simulink model "kurtosis_single_channel_subblocks"  (R2012b)
settings: Solver=ode45  StartTime=0.0  StopTime=3571  RelTol=1e-3
libraries: xbsIndex_r4 x454, xps_library x2, simulink_xsg_bridge x1
(part 1 of 4)
settings Model: Creator=sgowda  LastModifiedBy=sgowda

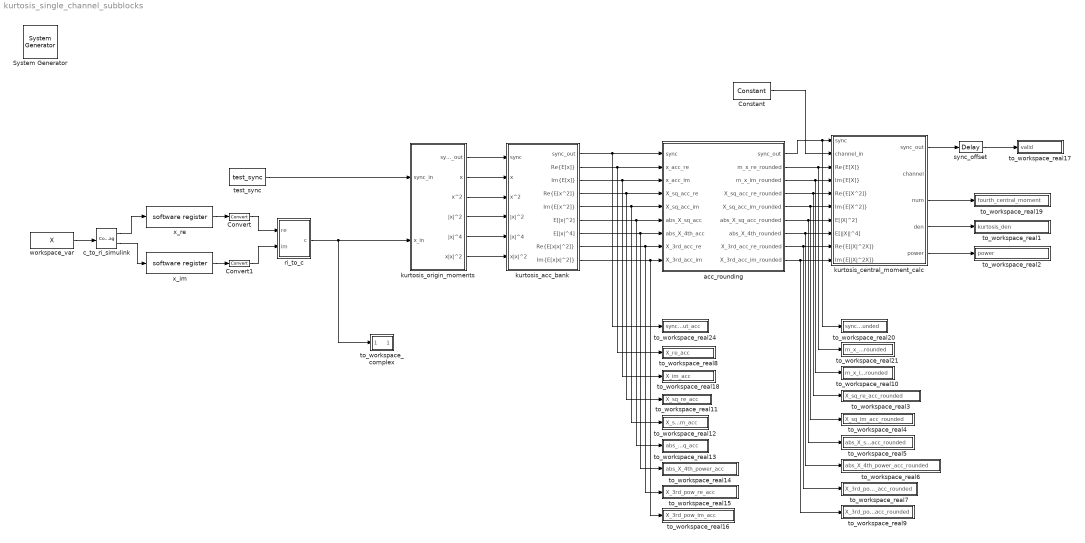
== system kurtosis_single_channel_subblocks ==
  " System Generator" : xbsIndex_r4/ System Generator  Tag=genX  xilinxfamily=Kintex7  part=xc7k325t  speed=-3  package=fbg676  synthesis_tool=XST  clock_wrapper=Clock Enables  directory=./netlist  proj_type=Project Navigator  Synth_file=XST Defaults  Impl_file=ISE Defaults  testbench=off  simulink_period=1  sysclk_period=10  dcm_input_clock_period=10  incr_netlist=off  trim_vbits=Everywhere in SubSystem  dbl_ovrd=According to Block Masks  core_generation=According to Block Masks  run_coregen=off  deprecated_control=off  eval_field=0  block_type=sysgen
  Constant : xbsIndex_r4/Constant  const=0  gui_display_data_type=Fixed-point  arith_type=Signed (2's comp)  n_bits=12  bin_pt=0  preci_type=Single  exp_width=8  frac_width=24  explicit_period=on  period=1  equ=P=C  opselect=C  inp2=PCIN>>17  opr=+  inp1=P  carry=CIN  dbl_ovrd=off  block_type=constant
  Convert : xbsIndex_r4/Convert  gui_display_data_type=Fixed-point  arith_type="Signed  (2's comp)"  n_bits=18  bin_pt=17  float_type=Single  exp_bits=8  fraction_bits=24  quantization=Truncate  overflow=Wrap  en=off  latency=0  dbl_ovrd=off  pipeline=off  block_type=convert
  Convert1 : xbsIndex_r4/Convert  gui_display_data_type=Fixed-point  arith_type="Signed  (2's comp)"  n_bits=18  bin_pt=17  float_type=Single  exp_bits=8  fraction_bits=24  quantization=Truncate  overflow=Wrap  en=off  latency=0  dbl_ovrd=off  pipeline=off  block_type=convert
  acc_rounding : Subsystem
  c_to_ri_simulink : ComplexToRealImag
  kurtosis_acc_bank : Subsystem
  kurtosis_central_moment_calc : Subsystem
  kurtosis_origin_moments : Subsystem
  ri_to_c : Subsystem
  sync_offset : xbsIndex_r4/Delay  rst=off  infoeditControl=Selection of Reset will increase slice count due to use of real FFs and instead of SRLs  en=off  latency=1  dbl_ovrd=off  reg_retiming=off  block_type=delay
  test_sync : simulink_xsg_bridge/test_sync
  to_workspace_complex : Subsystem  mask{var_name=X_fi, n_bits=18, bin_pt=17}
      mask prompts: var_name "Workspace variable name"; n_bits "# of bits"; bin_pt "Binary Point"
      mask init:
      | config.source = str2func('mat_output_data_cplx_init_xblock');
      | config.toplevel = gcb();
      | xBlock(config, {config.toplevel, 'var_name', var_name, ...
      |     'n_bits', n_bits, 'bin_pt', bin_pt});
  to_workspace_real1 : Subsystem  mask{var_name=kurtosis_den}
      mask prompts: var_name "Workspace variable name"
      mask init:
      | %config.source = str2func('mat_output_data_init_xblock');
      | %config.toplevel = gcb();
      | %xBlock(config, {config.toplevel, 'var_name', var_name});
  to_workspace_real10 : Subsystem  mask{var_name=m_x_im_rounded}
      mask prompts: var_name "Workspace variable name"
      mask init:
      | config.source = str2func('mat_output_data_init_xblock');
      | config.toplevel = gcb();
      | xBlock(config, {config.toplevel, 'var_name', var_name});
  to_workspace_real11 : Subsystem  mask{var_name=X_sq_re_acc}
      mask prompts: var_name "Workspace variable name"
      mask init:
      | %config.source = str2func('mat_output_data_init_xblock');
      | %config.toplevel = gcb();
      | %xBlock(config, {config.toplevel, 'var_name', var_name});
  to_workspace_real12 : Subsystem  mask{var_name=X_sq_im_acc}
      mask prompts: var_name "Workspace variable name"
      mask init:
      | %config.source = str2func('mat_output_data_init_xblock');
      | %config.toplevel = gcb();
      | %xBlock(config, {config.toplevel, 'var_name', var_name});
  to_workspace_real13 : Subsystem  mask{var_name=abs_X_sq_acc}
      mask prompts: var_name "Workspace variable name"
      mask init:
      | config.source = str2func('mat_output_data_init_xblock');
      | config.toplevel = gcb();
      | xBlock(config, {config.toplevel, 'var_name', var_name});
  to_workspace_real14 : Subsystem  mask{var_name=abs_X_4th_power_acc}
      mask prompts: var_name "Workspace variable name"
      mask init:
      | %config.source = str2func('mat_output_data_init_xblock');
      | %config.toplevel = gcb();
      | %xBlock(config, {config.toplevel, 'var_name', var_name});
  to_workspace_real15 : Subsystem  mask{var_name=X_3rd_pow_re_acc}
      mask prompts: var_name "Workspace variable name"
      mask init:
      | %config.source = str2func('mat_output_data_init_xblock');
      | %config.toplevel = gcb();
      | %xBlock(config, {config.toplevel, 'var_name', var_name});
  to_workspace_real16 : Subsystem  mask{var_name=X_3rd_pow_im_acc}
      mask prompts: var_name "Workspace variable name"
      mask init:
      | %config.source = str2func('mat_output_data_init_xblock');
      | %config.toplevel = gcb();
      | %xBlock(config, {config.toplevel, 'var_name', var_name});
  to_workspace_real17 : Subsystem  mask{var_name=valid}
      mask prompts: var_name "Workspace variable name"
      mask init:
      | config.source = str2func('mat_output_data_init_xblock');
      | config.toplevel = gcb();
      | xBlock(config, {config.toplevel, 'var_name', var_name});
  to_workspace_real18 : Subsystem  mask{var_name=X_im_acc}
      mask prompts: var_name "Workspace variable name"
      mask init:
      | config.source = str2func('mat_output_data_init_xblock');
      | config.toplevel = gcb();
      | xBlock(config, {config.toplevel, 'var_name', var_name});
  to_workspace_real19 : Subsystem  mask{var_name=fourth_central_moment}
      mask prompts: var_name "Workspace variable name"
      mask init:
      | %config.source = str2func('mat_output_data_init_xblock');
      | %config.toplevel = gcb();
      | %xBlock(config, {config.toplevel, 'var_name', var_name});
  to_workspace_real2 : Subsystem  mask{var_name=power}
      mask prompts: var_name "Workspace variable name"
      mask init:
      | config.source = str2func('mat_output_data_init_xblock');
      | config.toplevel = gcb();
      | xBlock(config, {config.toplevel, 'var_name', var_name});
  to_workspace_real20 : Subsystem  mask{var_name=sync_out_acc_rounded}
      mask prompts: var_name "Workspace variable name"
      mask init:
      | config.source = str2func('mat_output_data_init_xblock');
      | config.toplevel = gcb();
      | xBlock(config, {config.toplevel, 'var_name', var_name});
  to_workspace_real21 : Subsystem  mask{var_name=m_x_re_rounded}
      mask prompts: var_name "Workspace variable name"
      mask init:
      | config.source = str2func('mat_output_data_init_xblock');
      | config.toplevel = gcb();
      | xBlock(config, {config.toplevel, 'var_name', var_name});
  to_workspace_real24 : Subsystem  mask{var_name=sync_out_acc}
      mask prompts: var_name "Workspace variable name"
      mask init:
      | config.source = str2func('mat_output_data_init_xblock');
      | config.toplevel = gcb();
      | xBlock(config, {config.toplevel, 'var_name', var_name});
  to_workspace_real3 : Subsystem  mask{var_name=X_sq_re_acc_rounded}
      mask prompts: var_name "Workspace variable name"
      mask init:
      | config.source = str2func('mat_output_data_init_xblock');
      | config.toplevel = gcb();
      | xBlock(config, {config.toplevel, 'var_name', var_name});
  to_workspace_real4 : Subsystem  mask{var_name=X_sq_im_acc_rounded}
      mask prompts: var_name "Workspace variable name"
      mask init:
      | config.source = str2func('mat_output_data_init_xblock');
      | config.toplevel = gcb();
      | xBlock(config, {config.toplevel, 'var_name', var_name});
  to_workspace_real5 : Subsystem  mask{var_name=abs_X_sq_acc_rounded}
      mask prompts: var_name "Workspace variable name"
      mask init:
      | config.source = str2func('mat_output_data_init_xblock');
      | config.toplevel = gcb();
      | xBlock(config, {config.toplevel, 'var_name', var_name});
  to_workspace_real6 : Subsystem  mask{var_name=abs_X_4th_power_acc_rounded}
      mask prompts: var_name "Workspace variable name"
      mask init:
      | config.source = str2func('mat_output_data_init_xblock');
      | config.toplevel = gcb();
      | xBlock(config, {config.toplevel, 'var_name', var_name});
  to_workspace_real7 : Subsystem  mask{var_name=X_3rd_pow_re_acc_rounded}
      mask prompts: var_name "Workspace variable name"
      mask init:
      | config.source = str2func('mat_output_data_init_xblock');
      | config.toplevel = gcb();
      | xBlock(config, {config.toplevel, 'var_name', var_name});
  to_workspace_real8 : Subsystem  mask{var_name=X_re_acc}
      mask prompts: var_name "Workspace variable name"
      mask init:
      | config.source = str2func('mat_output_data_init_xblock');
      | config.toplevel = gcb();
      | xBlock(config, {config.toplevel, 'var_name', var_name});
  to_workspace_real9 : Subsystem  mask{var_name=X_3rd_pow_im_acc_rounded}
      mask prompts: var_name "Workspace variable name"
      mask init:
      | config.source = str2func('mat_output_data_init_xblock');
      | config.toplevel = gcb();
      | xBlock(config, {config.toplevel, 'var_name', var_name});
  workspace_var : FromWorkspace  VariableName=X  SampleTime=0
  x_im : xps_library/software register  Tag=xps:sw_reg  io_dir=From Processor  arith_type="Signed  (2's comp)"  bitwidth=32  bin_pt=17  sample_period=1  gw_name=kurtosis_single_channel_subblocks_x_im_user_data_out
      link override kurtosis_moment_calc_x_im_user_data_out: arith_type="Signed  (2's comp)"  n_bits=32  bin_pt=17  period=1
      link override untitled3_x_im_user_data_out: gui_display_data_type=Fixed-point  arith_type=Unsigned  n_bits=32  bin_pt=17  preci_type=Single  exp_width=8  frac_width=24  quantization=Truncate  overflow=Wrap  period=1  dbl_ovrd=off  timing_constraint=None  locs_specified=off  LOCs={}  UseAsADC=off  ADCChannel='1'  inherit_from_input=off  hdl_port=on
      link override untitled3_x_im_user_data_out: infoedit="Gateway in block.  Converts inputs of type Simulink integer, single, double and fixed-point to  Xilinx fixed-point or floating-point data type.<br><br>Hardware notes:  In hardware these blocks become top level input ports."
  x_re : xps_library/software register  Tag=xps:sw_reg  io_dir=From Processor  arith_type="Signed  (2's comp)"  bitwidth=32  bin_pt=17  sample_period=1  gw_name=kurtosis_single_channel_subblocks_x_re_user_data_out
      link override untitled3_x_re_user_data_out: gui_display_data_type=Fixed-point  arith_type="Signed  (2's comp)"  n_bits=32  bin_pt=17  preci_type=Single  exp_width=8  frac_width=24  quantization=Truncate  overflow=Wrap  period=1  dbl_ovrd=off  timing_constraint=None  locs_specified=off  LOCs={}  UseAsADC=off  ADCChannel='1'  inherit_from_input=off  hdl_port=on
      link override untitled3_x_re_user_data_out: infoedit="Gateway in block.  Converts inputs of type Simulink integer, single, double and fixed-point to  Xilinx fixed-point or floating-point data type.<br><br>Hardware notes:  In hardware these blocks become top level input ports."
  wires:
  kurtosis_central_moment_calc/1(sync_out) -> sync_offset/1
  sync_offset/1 -> to_workspace_real17/1(valid)
  kurtosis_acc_bank/2("Re{E[x]}") -> to_workspace_real8/1(X_re_acc), acc_rounding/2(x_acc_re)
  kurtosis_acc_bank/3("Im{E[x]}") -> to_workspace_real18/1(X_im_acc), acc_rounding/3(x_acc_im)
  kurtosis_acc_bank/4("Re{E[x^2]}") -> acc_rounding/4(X_sq_acc_re), to_workspace_real11/1(X_sq_re_acc)
  kurtosis_acc_bank/5("Im{E[x^2]}") -> acc_rounding/5(X_sq_acc_im), to_workspace_real12/1(X_sq_im_acc)
  kurtosis_acc_bank/6(E[|x|^2]) -> acc_rounding/6(abs_X_sq_acc), to_workspace_real13/1(abs_X_sq_acc)
  kurtosis_acc_bank/8("Re{E[x|x|^2]}") -> acc_rounding/8(X_3rd_acc_re), to_workspace_real15/1(X_3rd_pow_re_acc)
  kurtosis_acc_bank/7(E[|x|^4]) -> acc_rounding/7(abs_X_4th_acc), to_workspace_real14/1(abs_X_4th_power_acc)
  ri_to_c/1(c) -> kurtosis_origin_moments/2(x_in), to_workspace_complex/1(X_fi)
  Convert/1 -> ri_to_c/1(re)
  Convert1/1 -> ri_to_c/2(im)
  x_im/1 -> Convert1/1
  x_re/1 -> Convert/1
  workspace_var/1 -> c_to_ri_simulink/1
  c_to_ri_simulink/1 -> x_re/1
  c_to_ri_simulink/2 -> x_im/1
  kurtosis_acc_bank/9("Im{E[x|x|^2]}") -> acc_rounding/9(X_3rd_acc_im), to_workspace_real16/1(X_3rd_pow_im_acc)
  kurtosis_acc_bank/1(sync_out) -> acc_rounding/1(sync), to_workspace_real24/1(sync_out_acc)
  test_sync/1 -> kurtosis_origin_moments/1(sync_in)
  kurtosis_origin_moments/1(sync_out) -> kurtosis_acc_bank/1(sync)
  kurtosis_origin_moments/2(x) -> kurtosis_acc_bank/2(x)
  kurtosis_origin_moments/3(x^2) -> kurtosis_acc_bank/3(x^2)
  kurtosis_origin_moments/4(|x|^2) -> kurtosis_acc_bank/4(|x|^2)
  kurtosis_origin_moments/5(|x|^4) -> kurtosis_acc_bank/5(|x|^4)
  kurtosis_origin_moments/6(x|x|^2) -> kurtosis_acc_bank/6(x|x|^2)
  acc_rounding/1(sync_out) -> to_workspace_real20/1(sync_out_acc_rounded), kurtosis_central_moment_calc/1(sync)
  acc_rounding/9(X_3rd_acc_im_rounded) -> kurtosis_central_moment_calc/10("Im{E[|X|^2X]}"), to_workspace_real9/1(X_3rd_pow_im_acc_rounded)
  acc_rounding/8(X_3rd_acc_re_rounded) -> to_workspace_real7/1(X_3rd_pow_re_acc_rounded), kurtosis_central_moment_calc/9("Re{E[|X|^2X]}")
  acc_rounding/7(abs_X_4th_rounded) -> to_workspace_real6/1(abs_X_4th_power_acc_rounded), kurtosis_central_moment_calc/8(E[||X||^4])
  acc_rounding/6(abs_X_sq_acc_rounded) -> to_workspace_real5/1(abs_X_sq_acc_rounded), kurtosis_central_moment_calc/7(E[|X|^2])
  acc_rounding/5(X_sq_acc_im_rounded) -> to_workspace_real4/1(X_sq_im_acc_rounded), kurtosis_central_moment_calc/6("Im{E[X^2]}")
  acc_rounding/4(X_sq_acc_re_rounded) -> to_workspace_real3/1(X_sq_re_acc_rounded), kurtosis_central_moment_calc/5("Re{E[X^2]}")
  acc_rounding/3(m_x_im_rounded) -> to_workspace_real10/1(m_x_im_rounded), kurtosis_central_moment_calc/4("Im{E[X]}")
  acc_rounding/2(m_x_re_rounded) -> to_workspace_real21/1(m_x_re_rounded), kurtosis_central_moment_calc/3("Re{E[X]}")
  Constant/1 -> kurtosis_central_moment_calc/2(channel_in)
  kurtosis_central_moment_calc/4(den) -> to_workspace_real1/1(kurtosis_den)
  kurtosis_central_moment_calc/3(num) -> to_workspace_real19/1(fourth_central_moment)
  kurtosis_central_moment_calc/5(power) -> to_workspace_real2/1(power)

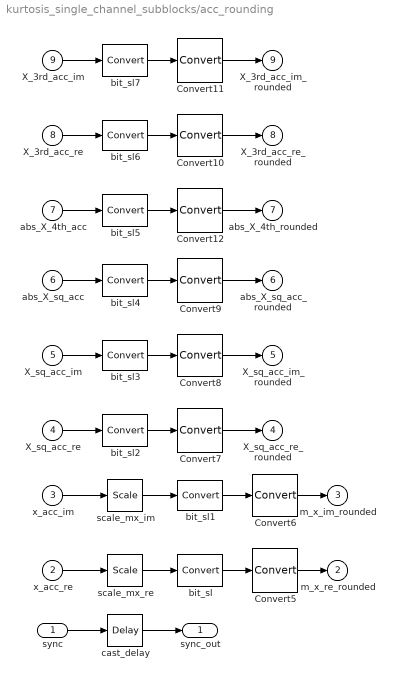
== system kurtosis_single_channel_subblocks/acc_rounding ==
  sync : Inport
  x_acc_re : Inport  Port=2
  x_acc_im : Inport  Port=3
  X_sq_acc_re : Inport  Port=4
  X_sq_acc_im : Inport  Port=5
  abs_X_sq_acc : Inport  Port=6
  abs_X_4th_acc : Inport  Port=7
  X_3rd_acc_re : Inport  Port=8
  X_3rd_acc_im : Inport  Port=9
  Convert{7..11} (5 alike) : xbsIndex_r4/Convert  gui_display_data_type=Fixed-point  arith_type="Signed  (2's comp)"  n_bits=35  bin_pt=22  float_type=Single  exp_bits=8  fraction_bits=24  quantization="Round  (unbiased: +/- Inf)"  overflow=Saturate  en=off  latency=5  dbl_ovrd=off  pipeline=off  block_type=convert
  Convert12 : xbsIndex_r4/Convert  gui_display_data_type=Fixed-point  arith_type="Signed  (2's comp)"  n_bits=84  bin_pt=68  float_type=Single  exp_bits=8  fraction_bits=24  quantization="Round  (unbiased: +/- Inf)"  overflow=Saturate  en=off  latency=5  dbl_ovrd=off  pipeline=off  block_type=convert
  Convert5 : xbsIndex_r4/Convert  gui_display_data_type=Fixed-point  arith_type="Signed  (2's comp)"  n_bits=25  bin_pt=24  float_type=Single  exp_bits=8  fraction_bits=24  quantization="Round  (unbiased: +/- Inf)"  overflow=Saturate  en=off  latency=5  dbl_ovrd=off  pipeline=off  block_type=convert
  Convert6 : xbsIndex_r4/Convert  gui_display_data_type=Fixed-point  arith_type="Signed  (2's comp)"  n_bits=25  bin_pt=24  float_type=Single  exp_bits=8  fraction_bits=24  quantization="Round  (unbiased: +/- Inf)"  overflow=Saturate  en=off  latency=5  dbl_ovrd=off  pipeline=off  block_type=convert
  bit_sl : xbsIndex_r4/Convert  gui_display_data_type=Fixed-point  arith_type="Signed  (2's comp)"  n_bits=28  bin_pt=27  float_type=Single  exp_bits=8  fraction_bits=24  quantization=Truncate  overflow=Wrap  en=off  latency=0  dbl_ovrd=off  pipeline=off  block_type=convert
  bit_sl1 : xbsIndex_r4/Convert  gui_display_data_type=Fixed-point  arith_type="Signed  (2's comp)"  n_bits=28  bin_pt=27  float_type=Single  exp_bits=8  fraction_bits=24  quantization=Truncate  overflow=Wrap  en=off  latency=0  dbl_ovrd=off  pipeline=off  block_type=convert
  bit_sl2 : xbsIndex_r4/Convert  gui_display_data_type=Fixed-point  arith_type="Signed  (2's comp)"  n_bits=47  bin_pt=34  float_type=Single  exp_bits=8  fraction_bits=24  quantization=Truncate  overflow=Wrap  en=off  latency=0  dbl_ovrd=off  pipeline=off  block_type=convert
  bit_sl3 : xbsIndex_r4/Convert  gui_display_data_type=Fixed-point  arith_type="Signed  (2's comp)"  n_bits=47  bin_pt=34  float_type=Single  exp_bits=8  fraction_bits=24  quantization=Truncate  overflow=Wrap  en=off  latency=0  dbl_ovrd=off  pipeline=off  block_type=convert
  bit_sl4 : xbsIndex_r4/Convert  gui_display_data_type=Fixed-point  arith_type="Signed  (2's comp)"  n_bits=47  bin_pt=34  float_type=Single  exp_bits=8  fraction_bits=24  quantization=Truncate  overflow=Wrap  en=off  latency=0  dbl_ovrd=off  pipeline=off  block_type=convert
  bit_sl5 : xbsIndex_r4/Convert  gui_display_data_type=Fixed-point  arith_type="Signed  (2's comp)"  n_bits=84  bin_pt=68  float_type=Single  exp_bits=8  fraction_bits=24  quantization=Truncate  overflow=Wrap  en=off  latency=0  dbl_ovrd=off  pipeline=off  block_type=convert
  bit_sl6 : xbsIndex_r4/Convert  gui_display_data_type=Fixed-point  arith_type="Signed  (2's comp)"  n_bits=64  bin_pt=51  float_type=Single  exp_bits=8  fraction_bits=24  quantization=Truncate  overflow=Wrap  en=off  latency=0  dbl_ovrd=off  pipeline=off  block_type=convert
  bit_sl7 : xbsIndex_r4/Convert  gui_display_data_type=Fixed-point  arith_type="Signed  (2's comp)"  n_bits=64  bin_pt=51  float_type=Single  exp_bits=8  fraction_bits=24  quantization=Truncate  overflow=Wrap  en=off  latency=0  dbl_ovrd=off  pipeline=off  block_type=convert
  cast_delay : xbsIndex_r4/Delay  rst=off  infoeditControl=Selection of Reset will increase slice count due to use of real FFs and instead of SRLs  en=off  latency=5  dbl_ovrd=off  reg_retiming=off  block_type=delay
  scale_mx_im : xbsIndex_r4/Scale  scale_factor=-10  dbl_ovrd=off  block_type=scale
  scale_mx_re : xbsIndex_r4/Scale  scale_factor=-10  dbl_ovrd=off  block_type=scale
  sync_out : Outport
  m_x_re_rounded : Outport  Port=2
  m_x_im_rounded : Outport  Port=3
  X_sq_acc_re_rounded : Outport  Port=4
  X_sq_acc_im_rounded : Outport  Port=5
  abs_X_sq_acc_rounded : Outport  Port=6
  abs_X_4th_rounded : Outport  Port=7
  X_3rd_acc_re_rounded : Outport  Port=8
  X_3rd_acc_im_rounded : Outport  Port=9
  wires:
  cast_delay/1 -> sync_out/1
  sync/1 -> cast_delay/1
  Convert11/1 -> X_3rd_acc_im_rounded/1
  bit_sl7/1 -> Convert11/1
  Convert10/1 -> X_3rd_acc_re_rounded/1
  bit_sl6/1 -> Convert10/1
  Convert12/1 -> abs_X_4th_rounded/1
  bit_sl5/1 -> Convert12/1
  Convert9/1 -> abs_X_sq_acc_rounded/1
  bit_sl4/1 -> Convert9/1
  Convert8/1 -> X_sq_acc_im_rounded/1
  bit_sl3/1 -> Convert8/1
  Convert7/1 -> X_sq_acc_re_rounded/1
  bit_sl2/1 -> Convert7/1
  Convert6/1 -> m_x_im_rounded/1
  bit_sl1/1 -> Convert6/1
  Convert5/1 -> m_x_re_rounded/1
  bit_sl/1 -> Convert5/1
  X_3rd_acc_im/1 -> bit_sl7/1
  X_3rd_acc_re/1 -> bit_sl6/1
  abs_X_4th_acc/1 -> bit_sl5/1
  abs_X_sq_acc/1 -> bit_sl4/1
  X_sq_acc_im/1 -> bit_sl3/1
  X_sq_acc_re/1 -> bit_sl2/1
  scale_mx_im/1 -> bit_sl1/1
  scale_mx_re/1 -> bit_sl/1
  x_acc_im/1 -> scale_mx_im/1
  x_acc_re/1 -> scale_mx_re/1

== system kurtosis_single_channel_subblocks/kurtosis_acc_bank ==
  sync : Inport
  x : Inport  Port=2
  x^2 : Inport  Port=3
  |x|^2 : Inport  Port=4
  |x|^4 : Inport  Port=5
  x|x|^2 : Inport  Port=6
  abs_x_4th_acc : Subsystem
  abs_x_sq_acc : Subsystem
  acc_rst : Subsystem
  x_acc : Subsystem
  x_cube_acc : Subsystem
  x_sq_acc : Subsystem
  sync_out : Outport
  "Re{E[x]}" : Outport  Port=2
  "Im{E[x]}" : Outport  Port=3
  "Re{E[x^2]}" : Outport  Port=4
  "Im{E[x^2]}" : Outport  Port=5
  E[|x|^2] : Outport  Port=6
  E[|x|^4] : Outport  Port=7
  "Re{E[x|x|^2]}" : Outport  Port=8
  "Im{E[x|x|^2]}" : Outport  Port=9
  wires:
  acc_rst/1(acc_rst) -> abs_x_4th_acc/1(sync), abs_x_sq_acc/1(sync), x_cube_acc/1(sync), x_sq_acc/1(sync), x_acc/1(sync)  "acc_rst"
  abs_x_4th_acc/1(+=b) -> E[|x|^4]/1
  |x|^4/1 -> abs_x_4th_acc/2(b)
  abs_x_sq_acc/1(+=b) -> E[|x|^2]/1
  |x|^2/1 -> abs_x_sq_acc/2(b)
  x_cube_acc/2(x_im_acc) -> "Im{E[x|x|^2]}"/1
  x_cube_acc/1(x_re_acc) -> "Re{E[x|x|^2]}"/1
  x|x|^2/1 -> x_cube_acc/2(x)
  x_sq_acc/2(x_im_acc) -> "Im{E[x^2]}"/1
  x_sq_acc/1(x_re_acc) -> "Re{E[x^2]}"/1
  x^2/1 -> x_sq_acc/2(x)
  x_acc/2(x_im_acc) -> "Im{E[x]}"/1
  x_acc/1(x_re_acc) -> "Re{E[x]}"/1
  x/1 -> x_acc/2(x)
  acc_rst/2(sync_out) -> sync_out/1
  sync/1 -> acc_rst/1(sync)

== system kurtosis_single_channel_subblocks/kurtosis_central_moment_calc ==
  sync : Inport
  channel_in : Inport  Port=2
  "Re{E[X]}" : Inport  Port=3
  "Im{E[X]}" : Inport  Port=4
  "Re{E[X^2]}" : Inport  Port=5
  "Im{E[X^2]}" : Inport  Port=6
  E[|X|^2] : Inport  Port=7
  E[||X||^4] : Inport  Port=8
  "Re{E[|X|^2X]}" : Inport  Port=9
  "Im{E[|X|^2X]}" : Inport  Port=10
  adder_tree_del : xbsIndex_r4/Convert  gui_display_data_type=Fixed-point  arith_type="Signed  (2's comp)"  n_bits=32  bin_pt=19  float_type=Single  exp_bits=8  fraction_bits=24  quantization="Round  (unbiased: +/- Inf)"  overflow=Saturate  en=off  latency=13  dbl_ovrd=off  pipeline=off  block_type=convert
  channel_del : xbsIndex_r4/Delay  rst=off  infoeditControl=Selection of Reset will increase slice count due to use of real FFs and instead of SRLs  en=off  latency=28  dbl_ovrd=off  reg_retiming=off  block_type=delay
  cross_product_del : xbsIndex_r4/Delay  rst=off  infoeditControl=Selection of Reset will increase slice count due to use of real FFs and instead of SRLs  en=off  latency=15  dbl_ovrd=off  reg_retiming=off  block_type=delay
  kurtosis_cross_products : Subsystem
  kurtosis_den : Subsystem
  kurtosis_num : Subsystem
  scale : xbsIndex_r4/Scale  scale_factor=-10  dbl_ovrd=off  block_type=scale
  sync_out : Outport
  channel : Outport  Port=2
  num : Outport  Port=3
  den : Outport  Port=4
  power : Outport  Port=5
  wires:
  E[|X|^2]/1 -> kurtosis_cross_products/6(E[|X|^2]), cross_product_del/1
  cross_product_del/1 -> kurtosis_den/1(E[|X|^2]), adder_tree_del/1
  channel_del/1 -> channel/1
  channel_in/1 -> channel_del/1
  kurtosis_num/2(E[|X-m_x|^4]) -> num/1
  kurtosis_num/1(sync_out) -> sync_out/1
  kurtosis_cross_products/9(|E[(x-mx)^2]|^2) -> kurtosis_num/8(|E[(x-mx)^2]|^2)
  kurtosis_cross_products/8(|m_x|^4) -> kurtosis_num/7(|m_x|^4)
  kurtosis_cross_products/6("Re{4E[X|X|^2*m_x]}") -> kurtosis_num/6("Re{4E[X|X|^2*m_x]}")
  kurtosis_cross_products/5("Re{2E[X^2*conj(m_x^2)]}") -> kurtosis_num/5("Re{2E[X^2*conj(m_x^2)]}")
  kurtosis_cross_products/4(E[|X|^4]) -> kurtosis_num/4(E[|X|^4])
  kurtosis_cross_products/3(4|m_x|^4) -> kurtosis_num/3(4|m_x|^4)
  kurtosis_cross_products/2(4E[|X|^2]|m_x|^2) -> kurtosis_num/2(4E[|X|^2]|m_x|^2)
  kurtosis_cross_products/1(sync_out) -> kurtosis_num/1(sync)
  kurtosis_den/1(E[|X-m_x|^2]^2) -> den/1
  kurtosis_cross_products/7(|m_x|^2) -> kurtosis_den/2(|m_x|^2)
  "Im{E[|X|^2X]}"/1 -> kurtosis_cross_products/9("Im{E[|X|^2X]}")
  "Re{E[|X|^2X]}"/1 -> kurtosis_cross_products/8("Re{E[|X|^2X]}")
  E[||X||^4]/1 -> kurtosis_cross_products/7(E[||X||^4])
  "Im{E[X^2]}"/1 -> kurtosis_cross_products/5("Im{E[X^2]}")
  "Re{E[X^2]}"/1 -> kurtosis_cross_products/4("Re{E[X^2]}")
  "Im{E[X]}"/1 -> kurtosis_cross_products/3("Im{E[X]}")
  "Re{E[X]}"/1 -> kurtosis_cross_products/2("Re{E[X]}")
  sync/1 -> kurtosis_cross_products/1(sync)
  scale/1 -> power/1
  adder_tree_del/1 -> scale/1

== system kurtosis_single_channel_subblocks/kurtosis_origin_moments ==
  sync_in : Inport
  x_in : Inport  Port=2
  abs_x_sq : Subsystem
  abs_x_sq_del : xbsIndex_r4/Delay  rst=off  infoeditControl=Selection of Reset will increase slice count due to use of real FFs and instead of SRLs  en=off  latency=5  dbl_ovrd=off  reg_retiming=off  block_type=delay
  c_to_ri_xin : Subsystem
  cplx_sq : Subsystem
  ri_to_c_x_3rd : Subsystem
  square_real : xbsIndex_r4/Mult  precision=Full  arith_type="Signed  (2's comp)"  n_bits=36  bin_pt=34  quantization=Truncate  overflow=Wrap  en=off  latency=5  dbl_ovrd=off  use_behavioral_HDL=off  opt=Speed  use_embedded=on  optimum_pipeline=off  pipeline=on  use_rpm=on  placement_style=Triangular  block_type=mult
  sync_delay : xbsIndex_r4/Delay  rst=off  infoeditControl=Selection of Reset will increase slice count due to use of real FFs and instead of SRLs  en=off  latency=10  dbl_ovrd=off  reg_retiming=off  block_type=delay
  third_power_im : xbsIndex_r4/Mult  precision=Full  arith_type="Signed  (2's comp)"  n_bits=36  bin_pt=34  quantization=Truncate  overflow=Wrap  en=off  latency=5  dbl_ovrd=off  use_behavioral_HDL=off  opt=Speed  use_embedded=on  optimum_pipeline=off  pipeline=on  use_rpm=on  placement_style=Triangular  block_type=mult
  third_power_re : xbsIndex_r4/Mult  precision=Full  arith_type="Signed  (2's comp)"  n_bits=36  bin_pt=34  quantization=Truncate  overflow=Wrap  en=off  latency=5  dbl_ovrd=off  use_behavioral_HDL=off  opt=Speed  use_embedded=on  optimum_pipeline=off  pipeline=on  use_rpm=on  placement_style=Triangular  block_type=mult
  x_delay : xbsIndex_r4/Delay  rst=off  infoeditControl=Selection of Reset will increase slice count due to use of real FFs and instead of SRLs  en=off  latency=10  dbl_ovrd=off  reg_retiming=off  block_type=delay
  x_im_del : xbsIndex_r4/Delay  rst=off  infoeditControl=Selection of Reset will increase slice count due to use of real FFs and instead of SRLs  en=off  latency=5  dbl_ovrd=off  reg_retiming=off  block_type=delay
  x_re_del : xbsIndex_r4/Delay  rst=off  infoeditControl=Selection of Reset will increase slice count due to use of real FFs and instead of SRLs  en=off  latency=5  dbl_ovrd=off  reg_retiming=off  block_type=delay
  x_sq_del : xbsIndex_r4/Delay  rst=off  infoeditControl=Selection of Reset will increase slice count due to use of real FFs and instead of SRLs  en=off  latency=4  dbl_ovrd=off  reg_retiming=off  block_type=delay
  sync_out : Outport
  x : Outport  Port=2
  x^2 : Outport  Port=3
  |x|^2 : Outport  Port=4
  |x|^4 : Outport  Port=5
  x|x|^2 : Outport  Port=6
  wires:
  x_in/1 -> c_to_ri_xin/1(c), abs_x_sq/1(c), cplx_sq/2(b), cplx_sq/1(a), x_delay/1
  abs_x_sq/1(power) -> third_power_im/2, third_power_re/2, square_real/2, square_real/1, abs_x_sq_del/1
  ri_to_c_x_3rd/1(c) -> x|x|^2/1
  third_power_im/1 -> ri_to_c_x_3rd/2(im)
  third_power_re/1 -> ri_to_c_x_3rd/1(re)
  x_im_del/1 -> third_power_im/1
  x_re_del/1 -> third_power_re/1
  c_to_ri_xin/2(im) -> x_im_del/1
  c_to_ri_xin/1(re) -> x_re_del/1
  square_real/1 -> |x|^4/1
  abs_x_sq_del/1 -> |x|^2/1
  x_sq_del/1 -> x^2/1
  cplx_sq/1(c) -> x_sq_del/1
  x_delay/1 -> x/1
  sync_delay/1 -> sync_out/1
  sync_in/1 -> sync_delay/1

== system kurtosis_single_channel_subblocks/ri_to_c ==
  re : Inport
  im : Inport  Port=2
  concat : xbsIndex_r4/Concat  num_inputs=2  dbl_ovrd=off  block_type=concat
  force_im : xbsIndex_r4/Reinterpret  force_arith_type=on  arith_type=Unsigned  force_bin_pt=on  bin_pt=0  block_type=reinterpret
  force_re : xbsIndex_r4/Reinterpret  force_arith_type=on  arith_type=Unsigned  force_bin_pt=on  bin_pt=0  block_type=reinterpret
  c : Outport
  wires:
  force_re/1 -> concat/1
  re/1 -> force_re/1
  force_im/1 -> concat/2
  im/1 -> force_im/1
  concat/1 -> c/1

== system kurtosis_single_channel_subblocks/to_workspace_complex ==
  X_fi : Inport
  c_to_ri : Subsystem
  imag_gateway : xbsIndex_r4/Gateway Out  inherit_from_input=on  hdl_port=off  timing_constraint=None  locs_specified=off  LOCs={}  UseAsDAC=off  DACChannel='1'  block_type=gatewayout
  real_gateway : xbsIndex_r4/Gateway Out  inherit_from_input=on  hdl_port=off  timing_constraint=None  locs_specified=off  LOCs={}  UseAsDAC=off  DACChannel='1'  block_type=gatewayout
  ri_to_c : RealImagToComplex
  workspace_output : ToWorkspace  VariableName=X_fi  SampleTime=-1
  _o : Outport
  wires:
  X_fi/1 -> c_to_ri/1(c), _o/1
  ri_to_c/1 -> workspace_output/1  "cplx"
  imag_gateway/1 -> ri_to_c/2
  real_gateway/1 -> ri_to_c/1
  c_to_ri/2(im) -> imag_gateway/1  "c_to_ri_out2"
  c_to_ri/1(re) -> real_gateway/1  "c_to_ri_out1"

== system kurtosis_single_channel_subblocks/to_workspace_real1 ==
  kurtosis_den : Inport
  gateway : xbsIndex_r4/Gateway Out  inherit_from_input=off  hdl_port=off  timing_constraint=None  locs_specified=off  LOCs={}  UseAsDAC=off  DACChannel='1'  block_type=gatewayout
  workspace_input : ToWorkspace  VariableName=kurtosis_den  SampleTime=-1
  wires:
  gateway/1 -> workspace_input/1
  kurtosis_den/1 -> gateway/1

== system kurtosis_single_channel_subblocks/to_workspace_real10 ==
  m_x_im_rounded : Inport
  gateway : xbsIndex_r4/Gateway Out  inherit_from_input=on  hdl_port=off  timing_constraint=None  locs_specified=off  LOCs={}  UseAsDAC=off  DACChannel='1'  block_type=gatewayout
  workspace_input : ToWorkspace  VariableName=m_x_im_rounded  SampleTime=-1
  wires:
  gateway/1 -> workspace_input/1
  m_x_im_rounded/1 -> gateway/1

== system kurtosis_single_channel_subblocks/to_workspace_real11 ==
  X_sq_re_acc : Inport
  gateway : xbsIndex_r4/Gateway Out  inherit_from_input=off  hdl_port=off  timing_constraint=None  locs_specified=off  LOCs={}  UseAsDAC=off  DACChannel='1'  block_type=gatewayout
  workspace_input : ToWorkspace  VariableName=X_sq_re_acc  SampleTime=-1
  wires:
  gateway/1 -> workspace_input/1
  X_sq_re_acc/1 -> gateway/1

== system kurtosis_single_channel_subblocks/to_workspace_real12 ==
  X_sq_im_acc : Inport
  gateway : xbsIndex_r4/Gateway Out  inherit_from_input=off  hdl_port=off  timing_constraint=None  locs_specified=off  LOCs={}  UseAsDAC=off  DACChannel='1'  block_type=gatewayout
  workspace_input : ToWorkspace  VariableName=X_sq_im_acc  SampleTime=-1
  wires:
  gateway/1 -> workspace_input/1
  X_sq_im_acc/1 -> gateway/1

== system kurtosis_single_channel_subblocks/to_workspace_real13 ==
  abs_X_sq_acc : Inport
  gateway : xbsIndex_r4/Gateway Out  inherit_from_input=on  hdl_port=off  timing_constraint=None  locs_specified=off  LOCs={}  UseAsDAC=off  DACChannel='1'  block_type=gatewayout
  workspace_input : ToWorkspace  VariableName=abs_X_sq_acc  SampleTime=-1
  wires:
  gateway/1 -> workspace_input/1
  abs_X_sq_acc/1 -> gateway/1

== system kurtosis_single_channel_subblocks/to_workspace_real14 ==
  abs_X_4th_power_acc : Inport
  gateway : xbsIndex_r4/Gateway Out  inherit_from_input=off  hdl_port=off  timing_constraint=None  locs_specified=off  LOCs={}  UseAsDAC=off  DACChannel='1'  block_type=gatewayout
  workspace_input : ToWorkspace  VariableName=abs_X_4th_power_acc  SampleTime=-1
  wires:
  gateway/1 -> workspace_input/1
  abs_X_4th_power_acc/1 -> gateway/1

== system kurtosis_single_channel_subblocks/to_workspace_real15 ==
  X_3rd_pow_re_acc : Inport
  gateway : xbsIndex_r4/Gateway Out  inherit_from_input=off  hdl_port=off  timing_constraint=None  locs_specified=off  LOCs={}  UseAsDAC=off  DACChannel='1'  block_type=gatewayout
  workspace_input : ToWorkspace  VariableName=X_3rd_pow_re_acc  SampleTime=-1
  wires:
  gateway/1 -> workspace_input/1
  X_3rd_pow_re_acc/1 -> gateway/1

== system kurtosis_single_channel_subblocks/to_workspace_real16 ==
  X_3rd_pow_im_acc : Inport
  gateway : xbsIndex_r4/Gateway Out  inherit_from_input=off  hdl_port=off  timing_constraint=None  locs_specified=off  LOCs={}  UseAsDAC=off  DACChannel='1'  block_type=gatewayout
  workspace_input : ToWorkspace  VariableName=X_3rd_pow_im_acc  SampleTime=-1
  wires:
  gateway/1 -> workspace_input/1
  X_3rd_pow_im_acc/1 -> gateway/1

== system kurtosis_single_channel_subblocks/to_workspace_real17 ==
  valid : Inport
  gateway : xbsIndex_r4/Gateway Out  inherit_from_input=on  hdl_port=off  timing_constraint=None  locs_specified=off  LOCs={}  UseAsDAC=off  DACChannel='1'  block_type=gatewayout
  workspace_input : ToWorkspace  VariableName=valid  SampleTime=-1
  wires:
  gateway/1 -> workspace_input/1
  valid/1 -> gateway/1

== system kurtosis_single_channel_subblocks/to_workspace_real18 ==
  X_im_acc : Inport
  gateway : xbsIndex_r4/Gateway Out  inherit_from_input=on  hdl_port=off  timing_constraint=None  locs_specified=off  LOCs={}  UseAsDAC=off  DACChannel='1'  block_type=gatewayout
  workspace_input : ToWorkspace  VariableName=X_im_acc  SampleTime=-1
  wires:
  gateway/1 -> workspace_input/1
  X_im_acc/1 -> gateway/1

== system kurtosis_single_channel_subblocks/to_workspace_real19 ==
  fourth_central_moment : Inport
  gateway : xbsIndex_r4/Gateway Out  inherit_from_input=off  hdl_port=off  timing_constraint=None  locs_specified=off  LOCs={}  UseAsDAC=off  DACChannel='1'  block_type=gatewayout
  workspace_input : ToWorkspace  VariableName=fourth_central_moment  SampleTime=-1
  wires:
  gateway/1 -> workspace_input/1
  fourth_central_moment/1 -> gateway/1

== system kurtosis_single_channel_subblocks/to_workspace_real2 ==
  power : Inport
  gateway : xbsIndex_r4/Gateway Out  inherit_from_input=on  hdl_port=off  timing_constraint=None  locs_specified=off  LOCs={}  UseAsDAC=off  DACChannel='1'  block_type=gatewayout
  workspace_input : ToWorkspace  VariableName=power  SampleTime=-1
  wires:
  gateway/1 -> workspace_input/1
  power/1 -> gateway/1

== system kurtosis_single_channel_subblocks/to_workspace_real20 ==
  sync_out_acc_rounded : Inport
  gateway : xbsIndex_r4/Gateway Out  inherit_from_input=on  hdl_port=off  timing_constraint=None  locs_specified=off  LOCs={}  UseAsDAC=off  DACChannel='1'  block_type=gatewayout
  workspace_input : ToWorkspace  VariableName=sync_out_acc_rounded  SampleTime=-1
  wires:
  gateway/1 -> workspace_input/1
  sync_out_acc_rounded/1 -> gateway/1

== system kurtosis_single_channel_subblocks/to_workspace_real21 ==
  m_x_re_rounded : Inport
  gateway : xbsIndex_r4/Gateway Out  inherit_from_input=on  hdl_port=off  timing_constraint=None  locs_specified=off  LOCs={}  UseAsDAC=off  DACChannel='1'  block_type=gatewayout
  workspace_input : ToWorkspace  VariableName=m_x_re_rounded  SampleTime=-1
  wires:
  gateway/1 -> workspace_input/1
  m_x_re_rounded/1 -> gateway/1

== system kurtosis_single_channel_subblocks/to_workspace_real24 ==
  sync_out_acc : Inport
  gateway : xbsIndex_r4/Gateway Out  inherit_from_input=on  hdl_port=off  timing_constraint=None  locs_specified=off  LOCs={}  UseAsDAC=off  DACChannel='1'  block_type=gatewayout
  workspace_input : ToWorkspace  VariableName=sync_out_acc  SampleTime=-1
  wires:
  gateway/1 -> workspace_input/1
  sync_out_acc/1 -> gateway/1

== system kurtosis_single_channel_subblocks/to_workspace_real3 ==
  X_sq_re_acc_rounded : Inport
  gateway : xbsIndex_r4/Gateway Out  inherit_from_input=on  hdl_port=off  timing_constraint=None  locs_specified=off  LOCs={}  UseAsDAC=off  DACChannel='1'  block_type=gatewayout
  workspace_input : ToWorkspace  VariableName=X_sq_re_acc_rounded  SampleTime=-1
  wires:
  gateway/1 -> workspace_input/1
  X_sq_re_acc_rounded/1 -> gateway/1

== system kurtosis_single_channel_subblocks/to_workspace_real4 ==
  X_sq_im_acc_rounded : Inport
  gateway : xbsIndex_r4/Gateway Out  inherit_from_input=on  hdl_port=off  timing_constraint=None  locs_specified=off  LOCs={}  UseAsDAC=off  DACChannel='1'  block_type=gatewayout
  workspace_input : ToWorkspace  VariableName=X_sq_im_acc_rounded  SampleTime=-1
  wires:
  gateway/1 -> workspace_input/1
  X_sq_im_acc_rounded/1 -> gateway/1

== system kurtosis_single_channel_subblocks/to_workspace_real5 ==
  abs_X_sq_acc_rounded : Inport
  gateway : xbsIndex_r4/Gateway Out  inherit_from_input=on  hdl_port=off  timing_constraint=None  locs_specified=off  LOCs={}  UseAsDAC=off  DACChannel='1'  block_type=gatewayout
  workspace_input : ToWorkspace  VariableName=abs_X_sq_acc_rounded  SampleTime=-1
  wires:
  gateway/1 -> workspace_input/1
  abs_X_sq_acc_rounded/1 -> gateway/1

== system kurtosis_single_channel_subblocks/to_workspace_real6 ==
  abs_X_4th_power_acc_rounded : Inport
  gateway : xbsIndex_r4/Gateway Out  inherit_from_input=on  hdl_port=off  timing_constraint=None  locs_specified=off  LOCs={}  UseAsDAC=off  DACChannel='1'  block_type=gatewayout
  workspace_input : ToWorkspace  VariableName=abs_X_4th_power_acc_rounded  SampleTime=-1
  wires:
  gateway/1 -> workspace_input/1
  abs_X_4th_power_acc_rounded/1 -> gateway/1

== system kurtosis_single_channel_subblocks/to_workspace_real7 ==
  X_3rd_pow_re_acc_rounded : Inport
  gateway : xbsIndex_r4/Gateway Out  inherit_from_input=on  hdl_port=off  timing_constraint=None  locs_specified=off  LOCs={}  UseAsDAC=off  DACChannel='1'  block_type=gatewayout
  workspace_input : ToWorkspace  VariableName=X_3rd_pow_re_acc_rounded  SampleTime=-1
  wires:
  gateway/1 -> workspace_input/1
  X_3rd_pow_re_acc_rounded/1 -> gateway/1

== system kurtosis_single_channel_subblocks/to_workspace_real8 ==
  X_re_acc : Inport
  gateway : xbsIndex_r4/Gateway Out  inherit_from_input=on  hdl_port=off  timing_constraint=None  locs_specified=off  LOCs={}  UseAsDAC=off  DACChannel='1'  block_type=gatewayout
  workspace_input : ToWorkspace  VariableName=X_re_acc  SampleTime=-1
  wires:
  gateway/1 -> workspace_input/1
  X_re_acc/1 -> gateway/1

== system kurtosis_single_channel_subblocks/to_workspace_real9 ==
  X_3rd_pow_im_acc_rounded : Inport
  gateway : xbsIndex_r4/Gateway Out  inherit_from_input=on  hdl_port=off  timing_constraint=None  locs_specified=off  LOCs={}  UseAsDAC=off  DACChannel='1'  block_type=gatewayout
  workspace_input : ToWorkspace  VariableName=X_3rd_pow_im_acc_rounded  SampleTime=-1
  wires:
  gateway/1 -> workspace_input/1
  X_3rd_pow_im_acc_rounded/1 -> gateway/1

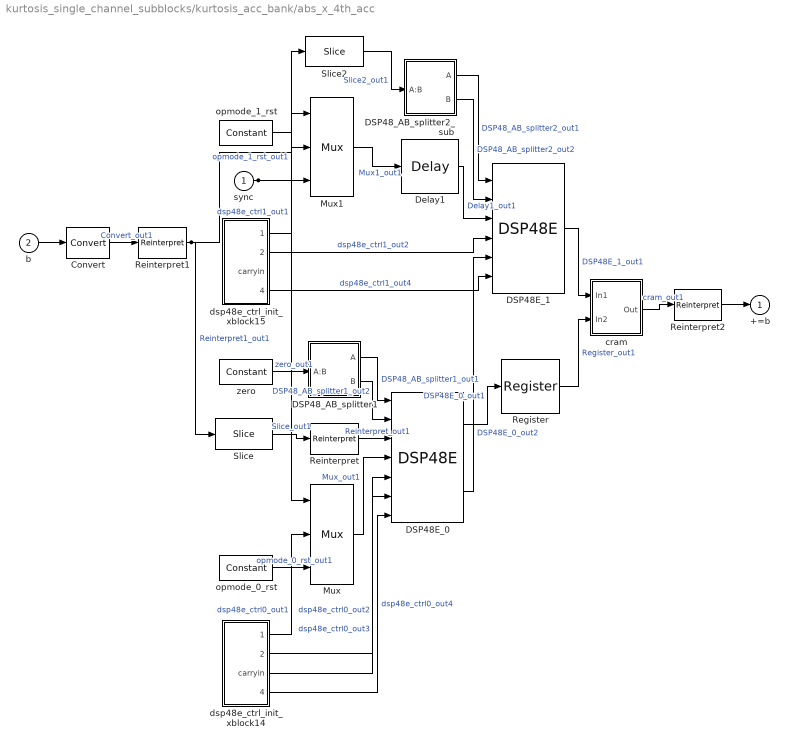
== system kurtosis_single_channel_subblocks/kurtosis_acc_bank/abs_x_4th_acc ==
  sync : Inport
  b : Inport  Port=2
  Convert : xbsIndex_r4/Convert  gui_display_data_type=Fixed-point  arith_type="Signed  (2's comp)"  n_bits=96  bin_pt=68  float_type=Single  exp_bits=8  fraction_bits=24  quantization=Truncate  overflow=Wrap  en=off  latency=0  dbl_ovrd=off  pipeline=off  block_type=convert
  DSP48E_0 : xbsIndex_r4/DSP48E  use_a=Direct from A Port  use_b=Direct from B Port  reset_preg=off  pattern_from_creg=on  pattern='000000000000'  mask_from_creg=on  pattern_mask='000000000000'  sel_rounding_mask=Select mask  use_op=off  use_creg=on  rst_all=off  en_all=off  use_pcin=off  use_carrycascin=off  use_multsignin=off  use_carryout=on  use_patterndetect=off  use_patternbdetect=off  use_overflow=off  use_underflow=off  use_acout=off  use_bcout=off  use_pcout=off  use_multsignout=off  use_carrycascout=off  pipeline_a=1  pipeline_b=1  pipeline_acout=1  pipeline_bcout=1  pipeline_c=on  pipeline_p=on  pipeline_mult=on  pipeline_opmode=on  pipeline_alumode=on  pipeline_carryin=on  pipeline_carryinsel=on  rst_a=off  rst_b=off  rst_c=off  rst_mult=off  rst_p=off  rst_carry_in=off  rst_alumode=off  rst_ctrl=off  en_a1=off  en_a2=off  en_b1=off  en_b2=off  en_c=off  en_mult=off  en_p=off  en_carry_in=off  en_alumode=off  en_multcarryin=off  en_ctrl=off  use_synth_model=off  addsub_mode=ONE48  xl_useadderonly=off  block_type=dsp48e
  DSP48E_1 : xbsIndex_r4/DSP48E  use_a=Direct from A Port  use_b=Direct from B Port  reset_preg=off  pattern_from_creg=on  pattern='000000000000'  mask_from_creg=on  pattern_mask='000000000000'  sel_rounding_mask=Select mask  use_op=off  use_creg=off  rst_all=off  en_all=off  use_pcin=off  use_carrycascin=off  use_multsignin=off  use_carryout=off  use_patterndetect=off  use_patternbdetect=off  use_overflow=off  use_underflow=off  use_acout=off  use_bcout=off  use_pcout=off  use_multsignout=off  use_carrycascout=off  pipeline_a=2  pipeline_b=2  pipeline_acout=1  pipeline_bcout=1  pipeline_c=on  pipeline_p=on  pipeline_mult=on  pipeline_opmode=on  pipeline_alumode=on  pipeline_carryin=off  pipeline_carryinsel=on  rst_a=off  rst_b=off  rst_c=off  rst_mult=off  rst_p=off  rst_carry_in=off  rst_alumode=off  rst_ctrl=off  en_a1=off  en_a2=off  en_b1=off  en_b2=off  en_c=off  en_mult=off  en_p=off  en_carry_in=off  en_alumode=off  en_multcarryin=off  en_ctrl=off  use_synth_model=off  addsub_mode=ONE48  xl_useadderonly=off  block_type=dsp48e
  DSP48_AB_splitter1 : Subsystem
  DSP48_AB_splitter2_sub : Subsystem
  Delay1 : xbsIndex_r4/Delay  rst=off  infoeditControl=Selection of Reset will increase slice count due to use of real FFs and instead of SRLs  en=off  latency=1  dbl_ovrd=off  reg_retiming=off  block_type=delay
  Mux : xbsIndex_r4/Mux  inputs=2  en=off  latency=0  precision=Full  arith_type=Unsigned  n_bits=16  bin_pt=14  quantization=Truncate  overflow=Wrap  dbl_ovrd=off  block_type=mux
  Mux1 : xbsIndex_r4/Mux  inputs=2  en=off  latency=0  precision=Full  arith_type=Unsigned  n_bits=16  bin_pt=14  quantization=Truncate  overflow=Wrap  dbl_ovrd=off  block_type=mux
  Register : xbsIndex_r4/Register  init=0  rst=off  en=off  dbl_ovrd=off  block_type=register
  Reinterpret : xbsIndex_r4/Reinterpret  force_arith_type=on  arith_type="Signed  (2's comp)"  force_bin_pt=on  bin_pt=0  block_type=reinterpret
  Reinterpret1 : xbsIndex_r4/Reinterpret  force_arith_type=on  arith_type="Signed  (2's comp)"  force_bin_pt=on  bin_pt=0  block_type=reinterpret
  Reinterpret2 : xbsIndex_r4/Reinterpret  force_arith_type=on  arith_type="Signed  (2's comp)"  force_bin_pt=on  bin_pt=68  block_type=reinterpret
  Slice : xbsIndex_r4/Slice  nbits=48  boolean_output=off  mode=Lower Bit Location + Width  bit1=0  base1=MSB of Input  bit0=0  base0=LSB of Input  dbl_ovrd=off  block_type=slice
  Slice2 : xbsIndex_r4/Slice  nbits=48  boolean_output=off  mode=Lower Bit Location + Width  bit1=0  base1=MSB of Input  bit0=48  base0=LSB of Input  dbl_ovrd=off  block_type=slice
  cram : Subsystem
  dsp48e_ctrl_init_xblock14 : Subsystem
  dsp48e_ctrl_init_xblock15 : Subsystem
  opmode_0_rst : xbsIndex_r4/Constant  const=12  gui_display_data_type=Fixed-point  arith_type=Unsigned  n_bits=7  bin_pt=0  preci_type=Single  exp_width=8  frac_width=24  explicit_period=on  period=1  equ=P=C  opselect=C  inp2=PCIN>>17  opr=+  inp1=P  carry=CIN  dbl_ovrd=off  block_type=constant
  opmode_1_rst : xbsIndex_r4/Constant  const=3  gui_display_data_type=Fixed-point  arith_type=Unsigned  n_bits=7  bin_pt=0  preci_type=Single  exp_width=8  frac_width=24  explicit_period=on  period=1  equ=P=C  opselect=C  inp2=PCIN>>17  opr=+  inp1=P  carry=CIN  dbl_ovrd=off  block_type=constant
  zero : xbsIndex_r4/Constant  const=0  gui_display_data_type=Fixed-point  arith_type=Signed (2's comp)  n_bits=48  bin_pt=0  preci_type=Single  exp_width=8  frac_width=24  explicit_period=on  period=1  equ=P=C  opselect=C  inp2=PCIN>>17  opr=+  inp1=P  carry=CIN  dbl_ovrd=off  block_type=constant
  +=b : Outport
  wires:
  sync/1 -> Mux1/1, Mux/1
  Reinterpret1/1 -> Slice2/1, Slice/1  "Reinterpret1_out1"
  dsp48e_ctrl_init_xblock15/4(carryinsel) -> DSP48E_1/6  "dsp48e_ctrl1_out4"
  dsp48e_ctrl_init_xblock15/2(alumode) -> DSP48E_1/4  "dsp48e_ctrl1_out2"
  dsp48e_ctrl_init_xblock15/1(opmode) -> Mux1/2  "dsp48e_ctrl1_out1"
  dsp48e_ctrl_init_xblock14/4(carryinsel) -> DSP48E_0/7  "dsp48e_ctrl0_out4"
  dsp48e_ctrl_init_xblock14/3(carryin) -> DSP48E_0/6  "dsp48e_ctrl0_out3"
  dsp48e_ctrl_init_xblock14/2(alumode) -> DSP48E_0/5  "dsp48e_ctrl0_out2"
  dsp48e_ctrl_init_xblock14/1(opmode) -> Mux/2  "dsp48e_ctrl0_out1"
  DSP48_AB_splitter2_sub/2(B) -> DSP48E_1/2  "DSP48_AB_splitter2_out2"
  DSP48_AB_splitter2_sub/1(A) -> DSP48E_1/1  "DSP48_AB_splitter2_out1"
  Slice2/1 -> DSP48_AB_splitter2_sub/1(A:B)  "Slice2_out1"
  zero/1 -> DSP48_AB_splitter1/1(A:B)  "zero_out1"
  opmode_1_rst/1 -> Mux1/3  "opmode_1_rst_out1"
  opmode_0_rst/1 -> Mux/3  "opmode_0_rst_out1"
  cram/1(Out) -> Reinterpret2/1  "cram_out1"
  Register/1 -> cram/2(In2)  "Register_out1"
  DSP48E_1/1 -> cram/1(In1)  "DSP48E_1_out1"
  Slice/1 -> Reinterpret/1  "Slice_out1"
  Reinterpret2/1 -> +=b/1
  Convert/1 -> Reinterpret1/1  "Convert_out1"
  Reinterpret/1 -> DSP48E_0/3  "Reinterpret_out1"
  DSP48E_0/1 -> Register/1  "DSP48E_0_out1"
  Mux1/1 -> Delay1/1  "Mux1_out1"
  Mux/1 -> DSP48E_0/4  "Mux_out1"
  Delay1/1 -> DSP48E_1/3  "Delay1_out1"
  DSP48_AB_splitter1/2(B) -> DSP48E_0/2  "DSP48_AB_splitter1_out2"
  DSP48_AB_splitter1/1(A) -> DSP48E_0/1  "DSP48_AB_splitter1_out1"
  DSP48E_0/2 -> DSP48E_1/5  "DSP48E_0_out2"
  b/1 -> Convert/1
